simulink model "modelo_f"  (R2024b)
settings: Solver=ode15s  StartTime=0.0  StopTime=inf  FixedStep=T_s  RelTol=1e-3
InitFcn:
  | clc
  | clear
  | close all
  | clear all
  | clear mex
  | parametros
  | gain_CL
  | calculo_observador_carro
  | calculo_observador_izaje
values from neighbouring files (symbols this model uses):
  b_cx = 1e6    (= 1000000)    [parametros.m]
  b_cy = 1e7    (= 10000000)    [parametros.m]
  b_hb = 1e8    (= 100000000)    [parametros.m]
  b_hd = 8    [parametros.m]
  b_hm = 18    [parametros.m]
  b_t = 90    [parametros.m]
  b_tb = 5e6    (= 5000000)    [parametros.m]
  b_td = 1.8    [parametros.m]
  b_tm = 6    [parametros.m]
  b_tw = 3e3    (= 3000)    [parametros.m]
  b_wu = 150    [parametros.m]
  container_pillars = container_pillars(randperm(19))    [parametros.m]
  dx_grid_lidar = 0.01    [parametros.m]
  escenario = 1    [parametros.m]
  g = 9.80665    [parametros.m]
  H_c = 2.59    [parametros.m]
  H_truck = 1    [parametros.m]
  i_h = 22    [parametros.m]
  i_t = 30    [parametros.m]
  J_hd_hEb = 3800    [parametros.m]
  J_hm_hb = 30    [parametros.m]
  J_td = 1200    [parametros.m]
  J_tm_tb = 7    [parametros.m]
  K_cy = 1.8e9    (= 1800000000)    [parametros.m]
  K_tw = 4.8e5    (= 480000)    [parametros.m]
  k_wu = 2.36e8    (= 236000000)    [parametros.m]
  l_h0 = (Y_t0-y_l0)    (= 38)    [parametros.m]
  l_h_max = Y_t0-y_h_min    (= 65)    [parametros.m]
  l_h_maxE = l_h_max+0.5    (= 65.5)    [parametros.m]
  l_h_min = Y_t0-y_h_max    (= 5)    [parametros.m]
  l_h_minE = l_h_min-0.5    (= 4.5)    [parametros.m]
  Lt = place(At', Ct', polos_deseados)'    [calculo_observador_carro.m]
  M_cmax = 50000    [parametros.m]
  M_cmin = 2000    [parametros.m]
  M_s = 15000    [parametros.m]
  M_t = 30000    [parametros.m]
  r_hd = 0.75    [parametros.m]
  r_td = 0.50    (= 0.5)    [parametros.m]
  T_hbMax = 5e4    (= 50000)    [parametros.m]
  T_hEbMax = 1.1e6    (= 1100000)    [parametros.m]
  T_hmMax = 2e4    (= 20000)    [parametros.m]
  T_s = 0.001    [parametros.m]
  T_s0 = 0.001    [parametros.m]
  T_s1 = 0.020    (= 0.02)    [parametros.m]
  T_s2 = 0.020    (= 0.02)    [parametros.m]
  T_tbMax = 5e3    (= 5000)    [parametros.m]
  T_tmMax = 4e3    (= 4000)    [parametros.m]
  tau_tm = 1e-3    (= 0.001)    [parametros.m]
  theta_hm0 = -l_h0*i_h*2/r_hd    (= -2229.33333333)    [parametros.m]
  theta_tm0 = (x_t0)*i_t/r_td    (= -900)    [parametros.m]
  trucks0 = [0, 0, 0, 0, 0]    [parametros.m]
  v_h_max_load = 1.5    [parametros.m]
  v_h_max_noload = 3    [parametros.m]
  v_lx0 = 0    [parametros.m]
  v_ly0 = 0    [parametros.m]
  v_t0 = 0    [parametros.m]
  v_t_max = 4    [parametros.m]
  W_c = ctrb(A, B_c(:,1))    [CyO_carro.m]    (also in CyO_izaje.m; parametros.m = 2.44)
  w_hm0 = 0    [parametros.m]
  w_hm_min_BRK = 0.005    [parametros.m]
  w_hm_rated = v_h_max_load*2*i_h/r_hd    (= 88)    [parametros.m]
  w_tm0 = (v_t0)*i_t/r_td    (= 0)    [parametros.m]
  w_tm_min_BRK = 0.005    [parametros.m]
  x_c0_left = -35    [parametros.m]
  x_c0_right = 55    [parametros.m]
  x_containers_left_lim = 1.5    [parametros.m]
  x_containers_right_lim = 48.5    [parametros.m]
  x_l0 = x_t0    (= -15)    [parametros.m]
  x_lidar_offset = 3.0    (= 3)    [parametros.m]
  x_t0 = -15    [parametros.m]
  x_t_max = 50    [parametros.m]
  x_t_maxE = x_t_max+0.5    (= 50.5)    [parametros.m]
  x_t_min = -30    [parametros.m]
  x_t_minE = x_t_min-0.5    (= -30.5)    [parametros.m]
  y_h_min = -20    [parametros.m]
  y_l0 = 7    [parametros.m]
  Y_sb = 5.0    (= 5)    [parametros.m]
  Y_t0 = 45    [parametros.m]
undefined symbols (not defined in the file or in its folder): Lh, parametros
libraries: dspnetwork x2, dspsigops x1, simulink x1
(part 3 of 4)

== matlab function modelo_f/UDP: Controller reader/MATLAB Function ==
  data: trolley_cmd output; hoist_cmd output; system_on output; twistlock output; sway_ctrl output; emergency output; emgy_ack output; data input
function [trolley_cmd, hoist_cmd, system_on, twistlock, sway_ctrl, emergency, emgy_ack] = parse_udp_packet(data)
% parse_udp_packet  Desempaqueta el datagrama de 13 bytes enviado por controller_reader.py
%
% Entrada:
%   data  : uint8(1x13) — bytes crudos del bloque UDP Receive
%
% Salidas (todas double):
%   trolley_cmd  [-4.0 .. +4.0] m/s   consigna velocidad carro
%   hoist_cmd    [-1.5 .. +1.5] m/s   consigna velocidad izaje
%   system_on    0/1   Sistema ON/OFF
%   twistlock    0/1   0=Abierto 1=Cerrado
%   sway_ctrl    0/1   Control de balanceo ON/OFF
%   emergency    0/1   Emergencia activa
%   emgy_ack     0/1   ACK de emergencia global
%
% Formato del paquete Python: struct.pack('!ffBBBBB', ...)
%   Big-endian: bytes 1-4 float32, 5-8 float32, 9-13 uint8
% -----------------------------------------------------------------------

% Valores por defecto (paquete malformado o vacío)
trolley_cmd = 0;
hoist_cmd   = 0;
system_on   = 0;
twistlock   = 0;
sway_ctrl   = 0;
emergency   = 0;
emgy_ack    = 0;

if numel(data) < 13
    return
end

raw = uint8(data(:)');   % forzar fila 1x13

% ── Floats big-endian → invertir bytes antes de typecast ──────────────
%    Python '!' = big-endian; x86/MATLAB = little-endian
trolley_cmd = double(typecast(raw(4:-1:1), 'single'));
hoist_cmd   = double(typecast(raw(8:-1:5), 'single'));

% ── Flags uint8 (un byte cada uno) ────────────────────────────────────
system_on = double(raw(9));
twistlock = double(raw(10));
sway_ctrl = double(raw(11));
emergency = double(raw(12));
emgy_ack  = double(raw(13));

== stateflow chart modelo_f/Nivel 0 - Seguridad y Protección ==
  state Safety_Security_Control
    entry:
    emgy = false;
    watchdog_fail = false;
    heartbeat_prev = false;
    hoist_solved = false;
    trolley_solved = false;
    state Emergencies [parallel]
      settings: executionOrder=1
      state Stand_By
        entry:
        hoist_solved = false;
        trolley_solved = false;
        emgy = false;
        during:
        BRK_hE = true;
        v_t_ref = v_t_ref_nvl_1;
        dl_h_ref = dl_h_ref_nvl_1;
        BRK_h = BRK_h_nvl_1;
        BRK_t = BRK_t_nvl_1;
        sway_ctr_enable = sway_ctr_enable_nvl_1;
        x_t_ref = x_t_ref_nvl_1;
      state Trolley_Emgy
        entry:
        trolley_emgy = true;
        BRK_t = false;
        trolley_solved = false;
        v_t_ref = 0;
        x_t_ref = x_t_estimada;
        state Init
        state Emgy_Switch_Min
          entry:
          BRK_t = true;
          during:
          v_t_ref = max([min([vx_joystick, 0.5]), 0]);
          dl_h_ref = vy_joystick;
        state Emgy_Switch_Max
          entry:
          BRK_t = true;
          during:
          v_t_ref = min([max([vx_joystick, -0.5]), 0]);
          dl_h_ref = vy_joystick;
        state Overspeed_Delay
        state Overspeed
          entry:
          sway_ctr_enable = false;
          state Init
          state Sway_Control
            entry:
            BRK_t = true;
            sway_ctr_enable = true;
          (default) -> Safety_Security_Control.Emergencies.Trolley_Emgy.Overspeed.Init
          Safety_Security_Control.Emergencies.Trolley_Emgy.Overspeed.Init -> Sway_Control : [after(3000, msec)]
        state Solved
          entry:
          trolley_emgy = false;
          trolley_solved = true;
        (default) -> Safety_Security_Control.Emergencies.Trolley_Emgy.Init
        Safety_Security_Control.Emergencies.Trolley_Emgy.Init -> Safety_Security_Control.Emergencies.Trolley_Emgy.Emgy_Switch_Min [order 1] : [FCE_carro_min && after(3000, msec)]
        Safety_Security_Control.Emergencies.Trolley_Emgy.Init -> Safety_Security_Control.Emergencies.Trolley_Emgy.Overspeed_Delay [order 3] : [sobrevelocidad_carro]
        Safety_Security_Control.Emergencies.Trolley_Emgy.Init -> Safety_Security_Control.Emergencies.Trolley_Emgy.Solved [order 4] : [after(10, sec)]
        Safety_Security_Control.Emergencies.Trolley_Emgy.Init -> Safety_Security_Control.Emergencies.Trolley_Emgy.Emgy_Switch_Max [order 2] : [FCE_carro_max && after(3000, msec)]
        Safety_Security_Control.Emergencies.Trolley_Emgy.Overspeed_Delay -> Safety_Security_Control.Emergencies.Trolley_Emgy.Overspeed : [after(3000, msec)]
        Safety_Security_Control.Emergencies.Trolley_Emgy.Emgy_Switch_Min -> Safety_Security_Control.Emergencies.Trolley_Emgy.Solved : [x_t_estimada >= x_t_safety_min]
        Safety_Security_Control.Emergencies.Trolley_Emgy.Emgy_Switch_Max -> Safety_Security_Control.Emergencies.Trolley_Emgy.Solved : [x_t_estimada <= x_t_safety_max]
        Safety_Security_Control.Emergencies.Trolley_Emgy.Overspeed -> Safety_Security_Control.Emergencies.Trolley_Emgy.Solved : [abs(theta_l*180/pi) <= 1]
      state Hoist_Emgy
        entry:
        hoist_emgy = true;
        BRK_hE = false;
        BRK_h = false;
        hoist_solved = false;
        dl_h_ref = 0;
        state Init
          during:
        state Emgy_Switch_Min
          entry:
          BRK_h = true;
          BRK_hE = true;
          during:
          v_t_ref = vx_joystick;
          dl_h_ref = max([min([vy_joystick, 0.5]), 0]);
        state Emgy_Switch_Max
          entry:
          BRK_h = true;
          BRK_hE = true;
          during:
          v_t_ref = vx_joystick;
          dl_h_ref = min([max([vy_joystick, -0.5]), 0]);
        state Overspeed_Delay
        state Overspeed
          entry:
          BRK_h = true;
          BRK_hE = true;
        state Solved
          entry:
          hoist_emgy = false;
          hoist_solved = true;
        (default) -> Safety_Security_Control.Emergencies.Hoist_Emgy.Init
        Safety_Security_Control.Emergencies.Hoist_Emgy.Init -> Safety_Security_Control.Emergencies.Hoist_Emgy.Emgy_Switch_Min [order 1] : [FCE_izaje_min && after(3000, msec)]
        Safety_Security_Control.Emergencies.Hoist_Emgy.Init -> Safety_Security_Control.Emergencies.Hoist_Emgy.Overspeed_Delay [order 3] : [sobrevelocidad_izaje]
        Safety_Security_Control.Emergencies.Hoist_Emgy.Init -> Safety_Security_Control.Emergencies.Hoist_Emgy.Solved [order 4] : [after(10, sec)]
        Safety_Security_Control.Emergencies.Hoist_Emgy.Init -> Safety_Security_Control.Emergencies.Hoist_Emgy.Emgy_Switch_Max [order 2] : [FCE_izaje_max && after(3000, msec)]
        Safety_Security_Control.Emergencies.Hoist_Emgy.Overspeed_Delay -> Safety_Security_Control.Emergencies.Hoist_Emgy.Overspeed : [after(3000, msec)]
        Safety_Security_Control.Emergencies.Hoist_Emgy.Emgy_Switch_Min -> Safety_Security_Control.Emergencies.Hoist_Emgy.Solved : [l_h >= l_h_safety_min]
        Safety_Security_Control.Emergencies.Hoist_Emgy.Emgy_Switch_Max -> Safety_Security_Control.Emergencies.Hoist_Emgy.Solved : [l_h <= l_h_safety_max]
        Safety_Security_Control.Emergencies.Hoist_Emgy.Overspeed -> Safety_Security_Control.Emergencies.Hoist_Emgy.Solved : [after(500, msec)]
      state Waiting_Global_Emgy_Ack
      state Global_Emgy
        entry:
        BRK_hE = false;
        BRK_t = false;
        BRK_h = false;
        emgy = true;
        sway_ctr_enable = false;
        during:
        v_t_ref = 0;
        dl_h_ref = 0;
      (default) -> Stand_By
      Stand_By -> Trolley_Emgy [order 3] : [FCE_carro_max || FCE_carro_min || sobrevelocidad_carro]
      Stand_By -> Global_Emgy [order 1] : [cmd_emgy_stop || watchdog_fail]
      Waiting_Global_Emgy_Ack -> Stand_By : [cmd_global_emgy_ack]{emgy=false;}
      Trolley_Emgy -> Stand_By : [trolley_solved]
      Stand_By -> Hoist_Emgy [order 2] : [FCE_izaje_min || FCE_izaje_max || sobrevelocidad_izaje]
      Hoist_Emgy -> Stand_By : [hoist_solved]
      Global_Emgy -> Waiting_Global_Emgy_Ack : [after(3000,msec)]
    state Watchdog [parallel]
      entry:
      counter = 0;
      heartbeat_prev = true;
      settings: executionOrder=2
      state Increase_counter
        entry:
        counter = counter + 1;
      state Init
      state Watchdog_Emgy
        entry:
        watchdog_fail = true;
      state Reset_Counter
        entry:
        counter = 0;
        heartbeat_prev = heartbeat;
      (default) -> Safety_Security_Control.Watchdog.Init
      Increase_counter -> Safety_Security_Control.Watchdog.Init
      Safety_Security_Control.Watchdog.Init -> Watchdog_Emgy [order 2] : [counter >= 5]
      Safety_Security_Control.Watchdog.Init -> Increase_counter [order 3] : [after(200, msec)]
      Safety_Security_Control.Watchdog.Init -> Reset_Counter [order 1] : [heartbeat_prev ~= heartbeat]
      Reset_Counter -> Safety_Security_Control.Watchdog.Init
  (default) -> Safety_Security_Control
  data: watchdog_fail local boolean size=1; counter local int8; heartbeat_prev local boolean; FCE_izaje_max input; FCE_carro_min input; FCE_carro_max input; FCE_izaje_min input; theta_l input; sobrevelocidad_izaje input; sobrevelocidad_carro input; emgy output boolean size=1 =false; BRK_t output boolean; BRK_hE output boolean; BRK_h output boolean; hoist_solved local; sway_ctr_enable output; dl_h_ref output; v_t_ref output; trolley_solved local; cmd_global_emgy_ack input; cmd_emgy_stop input; l_h_safety_min constant double =l_h_safety_min; vx_joystick input; vy_joystick input; x_t_safety_max constant double =x_t_safety_max; l_h input; l_h_safety_max constant double =l_h_safety_max; x_t_safety_min constant double =x_t_safety_min; x_t_estimada input; trolley_emgy output; hoist_emgy output; BRK_h_nvl_1 input; dl_h_ref_nvl_1 input; BRK_t_nvl_1 input boolean size=1; v_t_ref_nvl_1 input; heartbeat input boolean; sway_ctr_enable_nvl_1 input; x_t_ref output; x_t_ref_nvl_1 input

== matlab function modelo_f/TEST ==
  data: t input; heartbeat output; FCE_carro_max output; FCE_carro_min output; FCE_izaje_max output; FCE_izaje_min output; sobrevelocidad_izaje output; sobrevelocidad_carro output; cmd_emgy_stop output; cmd_global_emgy_ack output; x_t_estimada output; l_h output; theta_l output
function [heartbeat, FCE_carro_max, FCE_carro_min, FCE_izaje_max, FCE_izaje_min, ...
          sobrevelocidad_izaje, sobrevelocidad_carro, cmd_emgy_stop, cmd_global_emgy_ack, ...
          x_t_estimada, l_h, theta_l] = test_loader(t)

% ============================================================
%  SELECCION DE TEST - habilitar solo uno
% ============================================================
TEST_normal          = true;
TEST_heartbeat_fail  = false; % OK
TEST_emgy_carro_max  = false; % OK
TEST_emgy_carro_min  = false; % OK
TEST_emgy_izaje_max  = false; % OK
TEST_emgy_izaje_min  = false; % OK
TEST_sobrevel_izaje  = false; % OK
TEST_sobrevel_carro  = false; % OK
TEST_emgy_stop       = true;

% ============================================================
%  VALORES BASE
% ============================================================
heartbeat            = logical(mod(floor(t / 0.2), 2));
FCE_carro_max        = false;
FCE_carro_min        = false;
FCE_izaje_max        = false;
FCE_izaje_min        = false;
sobrevelocidad_izaje = false;
sobrevelocidad_carro = false;
cmd_emgy_stop        = false;
cmd_global_emgy_ack  = false;
x_t_estimada         = 0.0;
l_h                  = 0.0;
theta_l              = 0.0;

% ============================================================
%  TEST_heartbeat_fail
% ============================================================
if TEST_heartbeat_fail
    if t > 5.0
        heartbeat = false;
    end
end

% ============================================================
%  TEST_emgy_carro_max
% ============================================================
if TEST_emgy_carro_max
    if t >= 2.0 && t < 10.0
        x_t_estimada  = 50.0;
        FCE_carro_max = true;
    elseif t >= 10.0
        x_t_estimada  = 40.0;
        FCE_carro_max = false;
    end
end

% ============================================================
%  TEST_emgy_carro_min
% ============================================================
if TEST_emgy_carro_min
    if t >= 2.0 && t < 10.0
        x_t_estimada  = -30.0;
        FCE_carro_min = true;
    elseif t >= 10.0
        x_t_estimada  = -20.0;
        FCE_carro_min = false;
    end
end

% ============================================================
%  TEST_emgy_izaje_max
% ============================================================
if TEST_emgy_izaje_max
    if t >= 2.0 && t < 10.0
        l_h           = 65.0;
        FCE_izaje_max = true;
    elseif t >= 10.0
        l_h           = 55.0;
        FCE_izaje_max = false;
    end
end

% ============================================================
%  TEST_emgy_izaje_min
% ============================================================
if TEST_emgy_izaje_min
    if t >= 2.0 && t < 10.0
        l_h           = 5.0;
        FCE_izaje_min = true;
    elseif t >= 10.0
        l_h           = 10.0;
        FCE_izaje_min = false;
    end
end

% ============================================================
%  TEST_sobrevel_izaje
% ============================================================
if TEST_sobrevel_izaje
    if (t >= 2.0 && t < 3.0) || (t >= 18.0 && t < 19.0)
        sobrevelocidad_izaje = true;
    end
end

% ============================================================
%  TEST_sobrevel_carro
% ============================================================
if TEST_sobrevel_carro
    if t >= 2.0 && t < 3.0
        sobrevelocidad_carro = true;
    end
end

% ============================================================
%  TEST_emgy_stop
% ============================================================
if TEST_emgy_stop
    if t >= 4.0 && t < 5.0
        cmd_emgy_stop = true;
    end
    if t >= 10.0
        cmd_global_emgy_ack = true;
    end
end

end

== matlab function modelo_f/Generador Trayectoria 2 ==
  data: t input; x_t_star output; x_actual input; x_final input; v_actual input; NEW_TRAJ input; v_t_star output; a_t_star output
function [x_t_star, v_t_star, a_t_star] = generador_trayectoria(t, x_actual, x_final, v_actual, NEW_TRAJ)
    % ---------------------------------------------------------------------
    % PARÁMETROS Y LÍMITES OPERATIVOS
    % ---------------------------------------------------------------------
    v_max_limite    = 4.0 * 0.9;  % [m/s]
    a_max_limite    = 0.8 * 0.9;  % [m/s^2]
    
    tol_posicion    = 0.01;       % [m] Tolerancia de objetivo (1 cm)
    MAX_RECALCULOS  = 5;          % Máximo de recálculos permitidos

    % ---------------------------------------------------------------------
    % ESTADO PERSISTENTE
    % ---------------------------------------------------------------------
    persistent x_inicial t_inicio t_a t_crucero t_total v_crucero d_a d_crucero ...
               dir inicializado num_recalculos a_max_eff t_a_decel a_decel_eff ...
               fase3_ajustada

    if isempty(inicializado)
        inicializado   = false;
        x_inicial      = x_actual;
        t_inicio       = t;
        t_a            = 0;
        t_crucero      = 0;
        t_total        = 0;
        v_crucero      = 0;
        d_a            = 0;
        d_crucero      = 0;
        dir            = 0;
        num_recalculos = 0;
        a_max_eff      = a_max_limite;
        t_a_decel      = 0;
        a_decel_eff    = a_max_limite;
        fase3_ajustada = false;
    end

    t_eff = t - t_inicio;

    % ---------------------------------------------------------------------
    % EVALUACIÓN DE REPLANIFICACIÓN (DISPARO INMEDIATO EN t_total)
    % ---------------------------------------------------------------------
    if NEW_TRAJ == 1
        solicitar_replan = true;
        num_recalculos   = 0;
    else
        error_pos        = abs(x_final - x_actual);
        % Se engancha la siguiente S-curve inmediatamente en t_total si no llegó
        solicitar_replan = (t_eff >= t_total) && ...
                           (error_pos > tol_posicion) && ...
                           (num_recalculos < MAX_RECALCULOS);
    end

    if solicitar_replan
        if NEW_TRAJ == 0
            num_recalculos = num_recalculos + 1;
        end

        x_inicial      = x_actual;
        t_inicio       = t;
        D              = abs(x_final - x_inicial);
        dir            = sign(x_final - x_inicial);
        fase3_ajustada = false;

        if D <= tol_posicion
            t_a = 0; t_crucero = 0; t_total = 0;
            v_crucero = 0; d_a = 0; d_crucero = 0;
            a_max_eff = 0;
        else
            % Escalado suave para distancias cortas (< 2 m)
            a_max_eff = a_max_limite;
            v_max_eff = v_max_limite;
            if D < 2.0 
                a_max_eff = max(a_max_limite * (D / 2.0), a_max_limite * 0.05);
                v_max_eff = max(v_max_limite * (D / 2.0), v_max_limite * 0.05);
            end

            t_a = (pi * v_max_eff) / (2 * a_max_eff);
            d_a = (v_max_eff * t_a) / 2;
            if 2 * d_a >= D
                v_pico    = sqrt((2 * a_max_eff * D) / pi);
                t_a       = (pi * v_pico) / (2 * a_max_eff);
                t_crucero = 0;
                v_crucero = v_pico;
                d_crucero = 0;
                d_a       = D / 2;
            else
                v_crucero = v_max_eff;
                d_crucero = D - 2 * d_a;
                t_crucero = d_crucero / v_crucero;
            end
            t_a_decel   = t_a;
            a_decel_eff = a_max_eff;
            t_total     = 2 * t_a + t_crucero;
        end
        inicializado = true;
        t_eff        = 0;
    end

    % ---------------------------------------------------------------------
    % AJUSTE DINÁMICO AL ENTRAR A DESACELERACIÓN (~75% DEL TIEMPO)
    % ---------------------------------------------------------------------
    if (t_eff >= (t_a + t_crucero)) && (t_eff < t_total) && ~fase3_ajustada
        d_restante = abs(x_final - x_actual);
        if d_restante > tol_posicion && v_crucero > 1e-4
            % Reajuste del tiempo de frenado para cubrir exactamente d_restante
            t_a_decel   = (2 * d_restante) / v_crucero;
            a_decel_eff = (pi * v_crucero) / (2 * max(t_a_decel, 1e-3));
            
            % Mantenemos la aceleración dentro de los límites de seguridad
            if a_decel_eff > a_max_limite
                a_decel_eff = a_max_limite;
                t_a_decel   = (pi * v_crucero) / (2 * a_decel_eff);
            end
            
            t_total = t_a + t_crucero + t_a_decel;
        end
        fase3_ajustada = true;
    end

    % ---------------------------------------------------------------------
    % EVALUACIÓN DEL PERFIL DE TRAYECTORIA (S-CURVE)
    % ---------------------------------------------------------------------
    if t_a == 0 && t_crucero == 0
        x_t_star = x_final;
        v_t_star = 0;
        a_t_star = 0;
    elseif t_eff < t_a
        % Fase 1: Aceleración
        a_t_star = a_max_eff * sin(pi * t_eff / t_a) * dir;
        v_t_star = (a_max_eff * t_a / pi) * (1 - cos(pi * t_eff / t_a)) * dir;
        x_t_star = x_inicial + ((a_max_eff * t_a / pi) * (t_eff - (t_a / pi) * sin(pi * t_eff / t_a))) * dir;
    elseif t_eff < (t_a + t_crucero)
        % Fase 2: Crucero
        t_fase2  = t_eff - t_a;
        a_t_star = 0;
        v_t_star = v_crucero * dir;
        x_t_star = x_inicial + d_a * dir + v_crucero * t_fase2 * dir;
    elseif t_eff < t_total
        % Fase 3: Desaceleración Adaptativa Suave
        t_fase3      = t_eff - (t_a + t_crucero);
        x_fase3_init = x_inicial + (d_a + d_crucero) * dir;
        
        a_t_star = -a_decel_eff * sin(pi * t_fase3 / t_a_decel) * dir;
        v_t_star = (v_crucero - (a_decel_eff * t_a_decel / pi) * (1 - cos(pi * t_fase3 / t_a_decel))) * dir;
        x_t_star = x_fase3_init + (v_crucero * t_fase3 - (a_decel_eff * t_a_decel / pi) * (t_fase3 - (t_a_decel / pi) * sin(pi * t_fase3 / t_a_decel))) * dir;
    else
        % Estado de Reposo en la Meta (sin saltos ni caídas)
        x_t_star = x_final;
        v_t_star = 0;
        a_t_star = 0;
    end
end

== matlab function modelo_f/Nivel 2/MATLAB Function5 ==
  data: x_t_ref input; v_t_ref output; x_hat input; v_t_ff input; v_td_hat input; v_max input
function v_t_ref = controlador_posicion(x_t_ref, x_hat, v_t_ff,v_td_hat, v_max)

    % Kp = 2;
    Kd = 0;
    Kp = .11;

    e_x = x_t_ref - x_hat;
    % e_v = v_t_ff - v_td_hat;

    % v_calculada = (Kp * e_x) + e_v* Kd;
    v_calculada = Kp * e_x  + v_t_ff* Kd;

    if v_calculada > v_max
        v_t_ref = v_max;
    elseif v_calculada < -v_max
        v_t_ref = -v_max;
    else
        v_t_ref = v_calculada;
    end
end

== matlab function modelo_f/Nivel 2/MATLAB Function6 ==
  data: dl_h_ref output; l_h_ref input; l_h_sensor input; dl_h_ff input; m_est input
function dl_h_ref = controlador_posicion(l_h_ref, l_h_sensor, dl_h_ff, m_est)

    Kp = 0.5;

    e_l_h = l_h_ref - l_h_sensor;

    dl_h_ref = Kp * e_l_h; %+ dl_h_ff;

    if m_est > 16000
        dl_h_ref = min([1.5, max([dl_h_ref, -1.5])]);
    else
        dl_h_ref = min([3, max([dl_h_ref, -3])]);
    end
end

== matlab function modelo_f/Generador Trayectoria ==
  data: t input; t_inicio input; x_t_star output; x_inicial input; x_final input; v_t_star output; a_t_star output
function [x_t_star, v_t_star, a_t_star] = generador_trayectoria(t, t_inicio, x_inicial, x_final)
    % ---------------------------------------------------------------------
    % LIMITES OPERATIVOS (Sección 3.3) - PERFIL EN "S" (Jerk Limitado)
    % ---------------------------------------------------------------------
    v_max_limite = 4.0; % [m/s]
    a_max_limite = 0.8; % [m/s^2]
    
    % ESCUDO DE ESPERA
    if t < t_inicio
        x_t_star = x_inicial;
        v_t_star = 0;
        a_t_star = 0;
        return;
    end
    
    t_eff = t - t_inicio;
    D = abs(x_final - x_inicial);
    dir = sign(x_final - x_inicial);
    
    if D == 0
        x_t_star = x_inicial;
        v_t_star = 0;
        a_t_star = 0;
        return;
    end
    
    % ---------------------------------------------------------------------
    % CALCULO DEL PERFIL SENOIDAL (S-Curve)
    % ---------------------------------------------------------------------
    % Tiempo y distancia teórica para aceleración senoidal completa
    t_a = (pi * v_max_limite) / (2 * a_max_limite);
    d_a = (v_max_limite * t_a) / 2;
    
    if 2 * d_a >= D
        % El trayecto es corto: No llega a velocidad crucero (Perfil campana)
        v_pico = sqrt((2 * a_max_limite * D) / pi);
        t_a = (pi * v_pico) / (2 * a_max_limite);
        t_crucero = 0;
        v_crucero = v_pico;
        d_crucero = 0;
        d_a = D / 2;
    else
        % El trayecto es largo: Perfil en "S" con tramo de crucero plano
        v_crucero = v_max_limite;
        d_crucero = D - 2 * d_a;
        t_crucero = d_crucero / v_crucero;
    end
    
    t_total = 2 * t_a + t_crucero;
    
    % ---------------------------------------------------------------------
    % ECUACIONES CINEMÁTICAS INTEGRADAS (Onda Seno)
    % ---------------------------------------------------------------------
    if t_eff < t_a
        % Fase 1: Aceleración Suave (Onda Seno)
        a_t_star = a_max_limite * sin(pi * t_eff / t_a) * dir;
        v_t_star = (a_max_limite * t_a / pi) * (1 - cos(pi * t_eff / t_a)) * dir;
        x_t_star = x_inicial + ((a_max_limite * t_a / pi) * (t_eff - (t_a / pi) * sin(pi * t_eff / t_a))) * dir;
        
    elseif t_eff < (t_a + t_crucero)
        % Fase 2: Velocidad Constante (Crucero)
        t_fase2 = t_eff - t_a;
        a_t_star = 0;
        v_t_star = v_crucero * dir;
        x_t_star = x_inicial + d_a * dir + v_crucero * t_fase2 * dir;
        
    elseif t_eff < t_total
        % Fase 3: Desaceleración Suave (Onda Seno invertida)
        t_fase3 = t_eff - (t_a + t_crucero);
        a_t_star = -a_max_limite * sin(pi * t_fase3 / t_a) * dir;
        v_t_star = (v_crucero - (a_max_limite * t_a / pi) * (1 - cos(pi * t_fase3 / t_a))) * dir;
        x_t_star = x_inicial + (d_a + d_crucero) * dir + (v_crucero * t_fase3 - (a_max_limite * t_a / pi) * (t_fase3 - (t_a / pi) * sin(pi * t_fase3 / t_a))) * dir;
        
    else
        % Fase 4: Destino
        x_t_star = x_final;
        v_t_star = 0;
        a_t_star = 0;
    end
end

== matlab function modelo_f/Nivel 2/MATLAB Function2 ==
  data: sway_ctr_gain input; theta_hm input; theta_l input; v_balanceo output; w_l input; w_hm_hat input; enable input
function v_balanceo = controlador_balanceo_torque(sway_ctr_gain, theta_hm, theta_l, w_l, w_hm_hat, enable)
    persistent g r_hd i_h DEG2RAD 

    if isempty(g)
        DEG2RAD = pi/180;
        g       = 9.8066;
        r_hd    = 0.75;
        i_h     = 22;
    end

    if ~enable
        v_balanceo = 0;
        return;
    end

    l      = theta_hm * (-r_hd)/(i_h*2);
    dl_dt  = w_hm_hat * (-r_hd)/(i_h*2);
    l_seg  = max(l, 0.1);
    th_sat = max(-80*DEG2RAD, min(80*DEG2RAD, theta_l));
    w_o    = sqrt(g / l_seg);
    K_do   = (2*w_o*l_seg - 2*dl_dt) / cos(th_sat);
    v_balanceo = K_do * theta_l;   

end

== matlab function modelo_f/MATLAB Function1 ==
  data: t input; l_h_star output; t_inicio input; l_inicial input; l_final input; masa_total input; dl_h_star output; ddl_h_star output
function [l_h_star, dl_h_star, ddl_h_star] = generador_trayectoria_izaje(t, t_inicio, l_inicial, l_final, masa_total)
    % ---------------------------------------------------------------------
    % CONSTANTES FISICAS Y OPERATIVAS DE IZAJE
    % ---------------------------------------------------------------------
    g = 9.80665;               
    P_const = 956150;          
    v_max_absoluta = 3.0;      
    a_max_limite = 0.75;       
    
    % Operación a potencia constante según carga actual
    v_potencia = P_const / (masa_total * g);
    v_max_limite = min(v_max_absoluta, v_potencia);
    
    if t < t_inicio
        l_h_star = l_inicial;
        dl_h_star = 0;
        ddl_h_star = 0;
        return;
    end
    
    t_eff = t - t_inicio;
    D = abs(l_final - l_inicial);
    dir = sign(l_final - l_inicial); 
    
    if D == 0
        l_h_star = l_inicial;
        dl_h_star = 0;
        ddl_h_star = 0;
        return;
    end
    
    % ---------------------------------------------------------------------
    % CALCULO DEL PERFIL CINEMATICO (Curva S con Jerk continuo: 1 - cos)
    % ---------------------------------------------------------------------
    % Tiempo para alcanzar la velocidad máxima con este perfil
    t_a = 2 * v_max_limite / a_max_limite;
    d_a = v_max_limite * t_a / 2;
    
    if 2 * d_a >= D
        % Perfil sin crucero (Triangular ultra-suavizado)
        v_pico = sqrt((D * a_max_limite) / 2);
        t_a = 2 * v_pico / a_max_limite;
        t_crucero = 0;
        v_crucero = v_pico;
        d_crucero = 0;
        d_a = D / 2;
    else
        % Perfil Trapezoidal ultra-suavizado
        v_crucero = v_max_limite;
        d_crucero = D - 2 * d_a;
        t_crucero = d_crucero / v_crucero;
    end
    
    t_total = 2 * t_a + t_crucero;
    
    % ---------------------------------------------------------------------
    % EVALUACION INSTANTANEA
    % ---------------------------------------------------------------------
    if t_eff < t_a
        % Fase 1: Aceleración Suave (Perfil campana 1-cos)
        ddl_h_star = (a_max_limite / 2) * (1 - cos(2 * pi * t_eff / t_a)) * dir;
        dl_h_star = (a_max_limite / 2) * (t_eff - (t_a / (2 * pi)) * sin(2 * pi * t_eff / t_a)) * dir;
        l_h_star = l_inicial + (a_max_limite / 2) * ((t_eff^2 / 2) + (t_a^2 / (4 * pi^2)) * (cos(2 * pi * t_eff / t_a) - 1)) * dir;
        
    elseif t_eff < (t_a + t_crucero)
        % Fase 2: Velocidad Constante de Crucero
        t_fase2 = t_eff - t_a;
        ddl_h_star = 0;
        dl_h_star = v_crucero * dir;
        l_h_star = l_inicial + d_a * dir + v_crucero * t_fase2 * dir;
        
    elseif t_eff < t_total
        % Fase 3: Desaceleración Suave (Campana invertida 1-cos)
        t_fase3 = t_eff - (t_a + t_crucero);
        ddl_h_star = -(a_max_limite / 2) * (1 - cos(2 * pi * t_fase3 / t_a)) * dir;
        dl_h_star = (v_crucero - (a_max_limite / 2) * (t_fase3 - (t_a / (2 * pi)) * sin(2 * pi * t_fase3 / t_a))) * dir;
        
        d_recorrida_fase3 = v_crucero * t_fase3 - (a_max_limite / 2) * ((t_fase3^2 / 2) + (t_a^2 / (4 * pi^2)) * (cos(2 * pi * t_fase3 / t_a) - 1));
        l_h_star = l_inicial + (d_a + d_crucero + d_recorrida_fase3) * dir;
        
    else
        % Fase 4: Posición final alcanzada
        l_h_star = l_final;
        dl_h_star = 0;
        ddl_h_star = 0;
    end
end

== matlab function modelo_f/Nivel 2/Subsistema físico/MATLAB Function ==
  data: x_c0_left input; y_c0_contacto output; x_c0_right input; Y_sb input; W_c input; y_h_min input; H_c input; x_lidar_offset input; x_l input; container_pillars input; TLK input; x_t input; trucks0 input; H_truck input; Ts input; rand_in input; escenario input; x_containers_left_lim input; x_containers_right_lim input; t_camion_transicion input; y_c0_lidar output; containers_pillars_state output size=1,19; trucks_state output; trucks_has_load output; carga_tomada output
function [y_c0_contacto, y_c0_lidar, containers_pillars_state, trucks_state, trucks_has_load, carga_tomada] = ...
    perfil_suelo(x_c0_left, x_c0_right, Y_sb, W_c, y_h_min, H_c, x_lidar_offset, x_l, ...
                 container_pillars, TLK, x_t, trucks0, H_truck, Ts, rand_in, escenario, ...
                 x_containers_left_lim, x_containers_right_lim, t_camion_transicion)

persistent n_containers x_grid2 tlk_prev dx_grid idx_posiciones
persistent trucks_state_p trucks_has_load_p idx_trucks lambda_truck grupo_camion
persistent idx_zona_min idx_zona_max
persistent truck_en_transicion truck_timer
persistent carga_tomada_p

% Declarar tamaño variable seguro para arreglos dinámicos persistentes
coder.varsize('x_grid2', [1, 10000], [false, true]);
coder.varsize('n_containers', [1, 10000], [false, true]);

%% Inicialización de perfil de contenedores
if isempty(n_containers)
    dx_grid = 0.01;
    x_grid2 = x_c0_left : dx_grid : x_c0_right;
    n_containers = zeros(1, length(x_grid2));
    tlk_prev     = false;
    
    % --- Limites de la zona valida de contenedores (nunca escribir fuera de esto) ---
    idx_zona_min = round((x_containers_left_lim - x_c0_left) / dx_grid) + 1;
    idx_zona_max = round((x_containers_right_lim - x_c0_left) / dx_grid) + 1;
    idx_zona_min = max(1, min(length(x_grid2), idx_zona_min));
    idx_zona_max = max(1, min(length(x_grid2), idx_zona_max));
    
    % --- Carga inicial de pilas (19 posiciones estáticas garantizadas 1x19) ---
    n_pilares = 19;
    x_posiciones = linspace(x_containers_left_lim, x_containers_right_lim, n_pilares);
    idx_posiciones = zeros(1, 19);
    medio_ancho_idx = round((W_c/2) / dx_grid);
    
    for k = 1:n_pilares
        idx_pos = round((x_posiciones(k) - x_c0_left) / dx_grid) + 1;
        idx_pos = max(1, min(length(x_grid2), idx_pos));
        idx_posiciones(k) = idx_pos;
        
        idx_ini = max([1, idx_pos - medio_ancho_idx, idx_zona_min]);
        idx_fin = min([length(x_grid2), idx_pos + medio_ancho_idx, idx_zona_max]);
        n_containers(idx_ini:idx_fin) = container_pillars(k);
    end
    
    % --- Inicialización de camiones ---
    x_trucks_left = [-25 -20 -15 -10 -5];
    idx_trucks = zeros(1, 5);
    for k = 1:5
        idx_t = round((x_trucks_left(k) - x_c0_left) / dx_grid) + 1;
        idx_trucks(k) = max(1, min(length(x_grid2), idx_t));
    end
    
    trucks_state_p      = double(trucks0(:)'); % Forzar dimensiones 1x5
    trucks_has_load_p   = zeros(1,5);
    lambda_truck        = -log(0.5) / 60;
    grupo_camion        = ones(1,5);
    truck_en_transicion = zeros(1,5);
    truck_timer         = zeros(1,5);
    carga_tomada_p      = false;
end

%% Índice más cercano a x_l (posición de la carga)
idx = round((x_l - x_c0_left) / dx_grid) + 1;
idx = max(1, min(length(x_grid2), idx));
medio_ancho_idx = round((W_c/2) / dx_grid);

% La ventana de escritura/lectura de la carga nunca invade fuera
% de la zona valida de contenedores (evita que se mezcle con Y_sb u otras zonas)
idx_ini_l = max([1, idx - medio_ancho_idx, idx_zona_min]);
idx_fin_l = min([length(x_grid2), idx + medio_ancho_idx, idx_zona_max]);

%% Flancos de TLK
tlk_bool      = logical(TLK);
flanco_bajada = tlk_prev && ~tlk_bool;   % Soltar carga (1 -> 0)
flanco_subida = ~tlk_prev && tlk_bool;   % Tomar carga (0 -> 1)
tlk_prev      = tlk_bool;

% carga_tomada refleja directamente si el spreader esta enganchado a algo
% (TLK activo).
if flanco_subida
    carga_tomada_p = true;
elseif flanco_bajada
    carga_tomada_p = false;
end
carga_tomada = carga_tomada_p;

%% Identificar si la carga está sobre la posición de un camión
W_trucks_idx = round((W_c/2) / dx_grid);
sobre_camion_k = 0;
for k = 1:5
    if abs(idx - idx_trucks(k)) <= W_trucks_idx && trucks_state_p(k) == 1
        sobre_camion_k = k;
        break;
    end
end

%% Manejo de escenarios
if escenario ~= 0
    switch escenario
        case 1
            grupo_camion = ones(1,5);     % Carga
        case 2
            grupo_camion = 2*ones(1,5);   % Descarga
        case 3
            grupo_camion = [2 2 1 1 1];   % Mixto
    end
end

if sobre_camion_k > 0 && escenario ~= 0
    k = sobre_camion_k;
    if flanco_subida && grupo_camion(k) == 1 && trucks_has_load_p(k) == 1
        % El camión libera la carga instantáneamente al spreader
        trucks_has_load_p(k) = 0; 
        
        % Se arma un timer. El camión VACÍO se retira recién después
        truck_en_transicion(k) = 1;
        truck_timer(k) = 0;
        
    elseif flanco_bajada && grupo_camion(k) == 2 && trucks_has_load_p(k) == 0
        % NUEVA CORRECCIÓN: Al depositar, el camión recibe la carga instantáneamente
        trucks_has_load_p(k) = 1; 
        
        % Inicia el timer. El camión (CON CARGA) se retirará después de t_camion_transicion
        truck_en_transicion(k) = 1;
        truck_timer(k) = 0;
    end
else
    % Solo modifica n_containers si la ventana de escritura cae dentro de la zona valida
    if idx_fin_l >= idx_ini_l
        
        % Buscar el pilar fijo más cercano a la posición de la carga
        [dist_min, pilar_cercano] = min(abs(idx - idx_posiciones));
        
        % Si la carga está sobre uno de los pilares del barco/patio (tolerancia de medio ancho)
        if dist_min <= medio_ancho_idx
            % Hacemos "snap" a los índices exactos con los que se inicializó ese pilar
            idx_centro = idx_posiciones(pilar_cercano);
            idx_ini_write = max([1, idx_centro - medio_ancho_idx, idx_zona_min]);
            idx_fin_write = min([length(x_grid2), idx_centro + medio_ancho_idx, idx_zona_max]);
        else
            % Si está depositando fuera de las zonas predefinidas (caída libre)
            idx_ini_write = idx_ini_l;
            idx_fin_write = idx_fin_l;
        end
        
        if flanco_bajada
            altura_actual = max(n_containers(idx_ini_write:idx_fin_write));
            n_containers(idx_ini_write:idx_fin_write) = max(n_containers(idx_ini_write:idx_fin_write), altura_actual + 1);
        elseif flanco_subida
            altura_actual = max(n_containers(idx_ini_write:idx_fin_write));
            n_containers(idx_ini_write:idx_fin_write) = max(0, altura_actual - 1);
        end
    end
end

%% Reaparición probabilística
if escenario ~= 0
    p_ciclo = 1 - exp(-lambda_truck * Ts);
    for k = 1:5
        if trucks_state_p(k) == 0
            if rand_in(k) < p_ciclo
                trucks_state_p(k) = 1;
                if grupo_camion(k) == 1
                    trucks_has_load_p(k) = 1;
                else
                    trucks_has_load_p(k) = 0;
                end
                truck_en_transicion(k) = 0; % camion nuevo, sin transicion pendiente
                truck_timer(k) = 0;
            end
        end
    end
end

%% Altura fija según zona
if x_l < -1
    y_fijo = 0;
elseif x_l >= -1 && x_l <= 0
    y_fijo = Y_sb;
else
    y_fijo = y_h_min;
end

%% Aporte de altura de camiones
h_truck_l = 0;
for k = 1:5
    if abs(idx - idx_trucks(k)) <= W_trucks_idx && trucks_state_p(k) == 1
        % Discriminar entre camión con carga y plataforma vacía
        if trucks_has_load_p(k) == 1
            h_truck_l = H_truck + H_c; % Altura con contenedor (activo durante los 30s de salida)
        else
            h_truck_l = H_truck;       % Altura solo de la plataforma
        end
    end
end

%% Altura total de contacto
if idx_fin_l >= idx_ini_l
    altura_containers_l = max(n_containers(idx_ini_l:idx_fin_l));
else
    altura_containers_l = 0;
end
y_c0_contacto = y_fijo + altura_containers_l * H_c + h_truck_l;

%% Resolucion de camiones en transicion (basado en TIEMPO)
% Cada camion en transicion incrementa su timer en cada paso; cuando
% supera t_camion_transicion segundos, recien ahi desaparece de verdad.
for k = 1:5
    if truck_en_transicion(k) == 1
        truck_timer(k) = truck_timer(k) + Ts;
        if truck_timer(k) >= t_camion_transicion
            trucks_state_p(k)      = 0;
            trucks_has_load_p(k)   = 0; % Limpia el camión y su carga
            truck_en_transicion(k) = 0;
            truck_timer(k)         = 0;
        end
    end
end

%% Lectura de Lidar
x_laser = x_t + x_lidar_offset;
idx_lidar = round((x_laser - x_c0_left) / dx_grid) + 1;
idx_lidar = max(1, min(length(x_grid2), idx_lidar));

if x_laser < -1
    y_fijo_lidar = 0;
elseif x_laser >= -1 && x_laser <= 0
    y_fijo_lidar = Y_sb;
else
    y_fijo_lidar = y_h_min;
end

h_truck_lidar = 0;
for k = 1:5
    if abs(idx_lidar - idx_trucks(k)) <= W_trucks_idx && trucks_state_p(k) == 1
        if trucks_has_load_p(k) == 1
            h_truck_lidar = H_truck + H_c;
        else
            h_truck_lidar = H_truck;
        end
    end
end
y_c0_lidar = y_fijo_lidar + n_containers(idx_lidar) * H_c + h_truck_lidar;

%% Salidas garantizadas
containers_pillars_state = n_containers(idx_posiciones);
trucks_state              = trucks_state_p;
trucks_has_load           = trucks_has_load_p;
end
